simulink model "Problem2"  (R2020a)
settings: Solver=VariableStepAuto  StartTime=0.0  StopTime=100.0  RelTol=1e-3
settings Model: Creator=HP  LastModifiedBy=HP

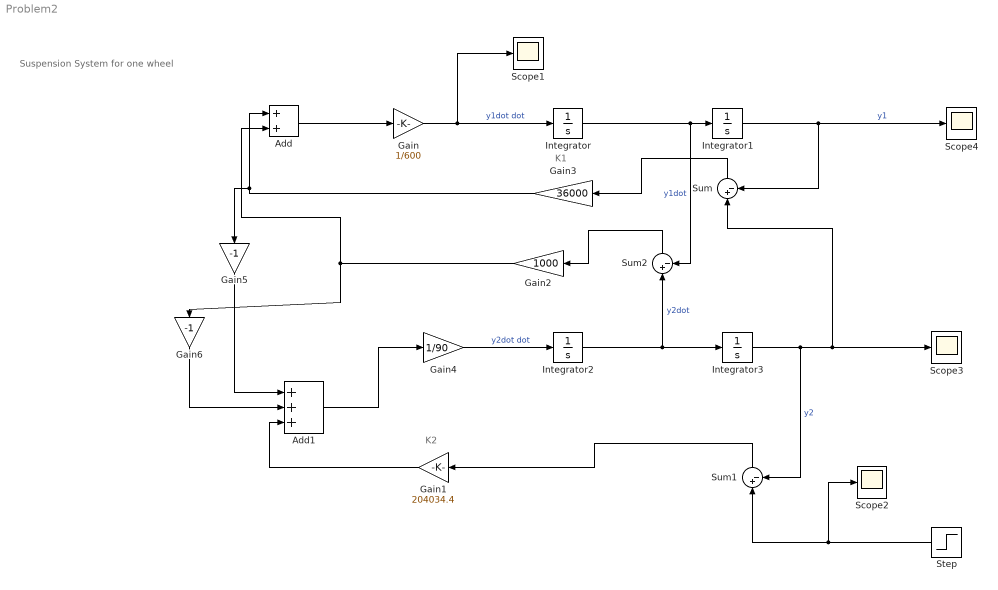
== system Problem2 ==
  note: K2
  note: K1
  note: Suspension System for one wheel
  Add : Sum
  Add1 : Sum  Inputs=+++
  Gain : Gain  Gain=1/600
  Gain1 : Gain  Gain=204034.4
  Gain2 : Gain  Gain=1000
  Gain3 : Gain  Gain=36000
  Gain4 : Gain  Gain=1/90
  Gain5 : Gain  Gain=-1
  Gain6 : Gain  Gain=-1
  Integrator{,1..3} (4 alike) : Integrator
  Scope{1..4} (4 alike) : Scope
  Step : Step  SampleTime=0
  Sum : Sum  Inputs=|+-
  Sum1 : Sum  Inputs=|+-
  Sum2 : Sum  Inputs=|+-
  wires:
  Gain1/1 -> Add1/3
  Sum1/1 -> Gain1/1
  Step/1 -> Scope2/1, Sum1/1
  Add1/1 -> Gain4/1
  Gain4/1 -> Integrator2/1  "y2dot dot"
  Integrator2/1 -> Sum2/1, Integrator3/1  "y2dot"
  Integrator3/1 -> Sum1/2, Sum/1, Scope3/1  "y2"
  Gain6/1 -> Add1/2
  Gain5/1 -> Add1/1
  Gain3/1 -> Gain5/1, Add/1
  Gain2/1 -> Gain6/1, Add/2
  Add/1 -> Gain/1
  Gain/1 -> Scope1/1, Integrator/1  "y1dot dot"
  Integrator/1 -> Integrator1/1, Sum2/2  "y1dot"
  Integrator1/1 -> Scope4/1, Sum/2  "y1"
  Sum/1 -> Gain3/1
  Sum2/1 -> Gain2/1
